simulink model "temperatura"  (R2021b)
settings: Solver=VariableStepAuto  StartTime=0.0  StopTime=30  RelTol=1e-3
settings Model: Creator=Voic  LastModifiedBy=Voic

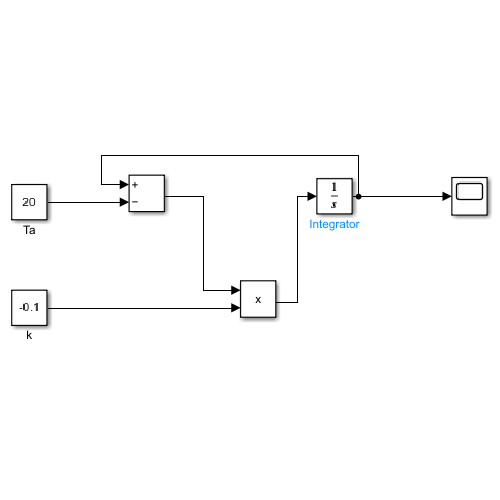
[thumbnail: Simulink's stored preview of the top-level diagram]
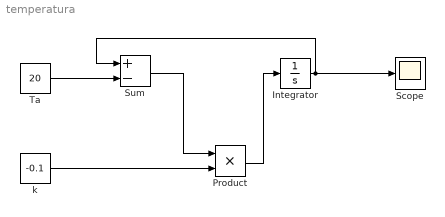
== system temperatura ==
  Integrator : Integrator  InitialCondition=60
  Product : Product
  Scope : Scope
  Sum : Sum  Inputs=+-
  Ta : Constant  Value=20
  k : Constant  Value=-0.1
  wires:
  Ta/1 -> Sum/2
  Integrator/1 -> Scope/1, Sum/1
  Product/1 -> Integrator/1
  k/1 -> Product/2
  Sum/1 -> Product/1
